simulink model "PathFollower"  (R2024b)
settings: Solver=VariableStepAuto  StartTime=0.0  StopTime=tsReplan  RelTol=1e-3
undefined symbols (not defined in the file or in its folder): gridLoc, mat, nRefPathRows, res
settings Model: Creator=cstabile  LastModifiedBy=jbrault
settings SolverCC: DateTimeAtSimulationTimeZero=[]
settings SFSimCC: SimTargetLang=C++
settings RTWCC: GPUComputeCapability=3.5

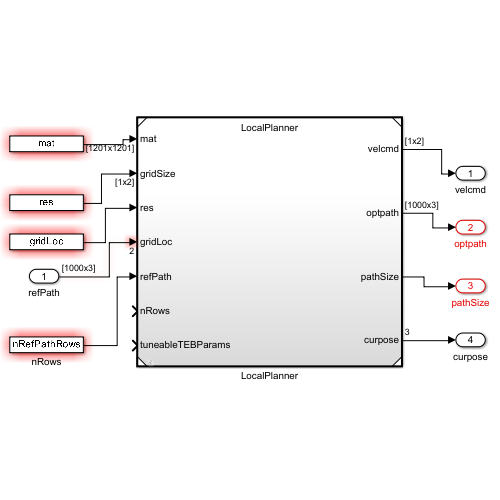
[thumbnail: Simulink's stored preview of the top-level diagram]
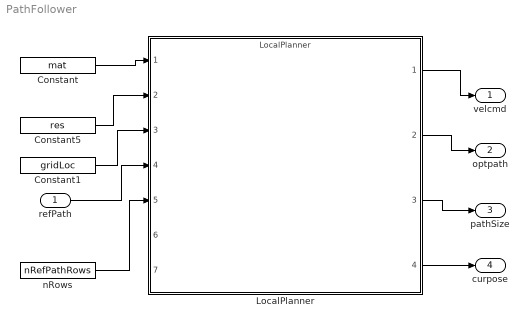
== system PathFollower ==
  refPath : Inport  PortDimensions=[1e3 3]  Interpolate=off
  Constant : Constant  Value=mat
  Constant1 : Constant  Value=gridLoc
  Constant5 : Constant  Value=res
  LocalPlanner : ModelReference  ModelNameDialog=LocalPlanner  SimulationMode=Normal  ModelReferenceVersion=2.0
  nRows : Constant  Value=nRefPathRows
  velcmd : Outport
  optpath : Outport  Port=2
  pathSize : Outport  Port=3
  curpose : Outport  Port=4
  wires:
  Constant/1 -> LocalPlanner/1
  Constant5/1 -> LocalPlanner/2
  Constant1/1 -> LocalPlanner/3
  refPath/1 -> LocalPlanner/4
  LocalPlanner/1 -> velcmd/1
  LocalPlanner/2 -> optpath/1
  LocalPlanner/3 -> pathSize/1
  LocalPlanner/4 -> curpose/1
  nRows/1 -> LocalPlanner/5
